simulink model "Scratch_Start"  (R2022a)
settings: Solver=VariableStepAuto  StartTime=0.0  StopTime=inf  RelTol=1e-3
libraries: robotlib x2, simulink x1
settings Model: Creator=dorleco  LastModifiedBy=dorleco

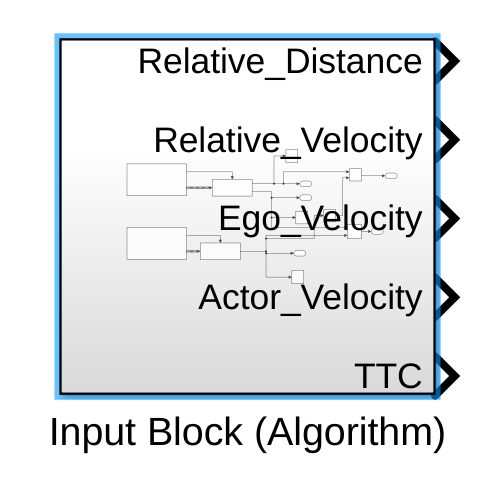
[thumbnail: Simulink's stored preview of the top-level diagram]
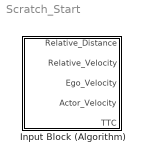
== system Scratch_Start ==
  Input Block (Algorithm) : Subsystem

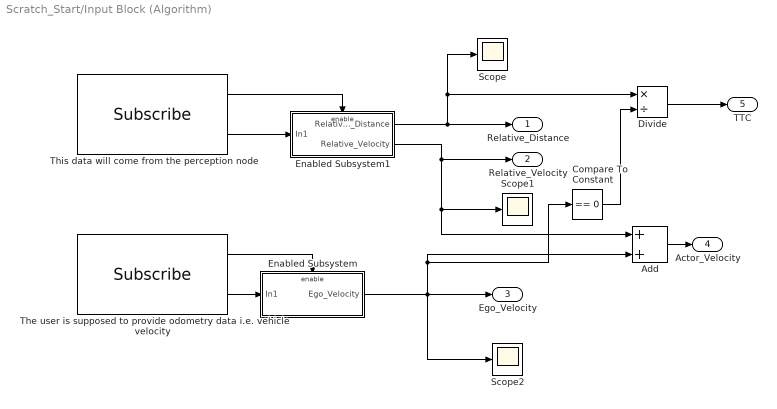
== system Scratch_Start/Input Block (Algorithm) ==
  Add : Sum
  Compare To Constant : simulink/Logic and Bit Operations/Compare To Constant  relop===  const=0  OutDataTypeStr=boolean
  Divide : Product  Inputs=*/
  Enabled Subsystem : Subsystem  TreatAsAtomicUnit=on
  Enabled Subsystem1 : Subsystem  TreatAsAtomicUnit=on
  Scope : Scope
  Scope1 : Scope
  Scope2 : Scope
  The user is supposed to provide odometry data i.e. vehicle velocity : robotlib/Subscribe  topicSource=Select from ROS network  topic=/carla/ego_vehicle/odometry  messageType=nav_msgs/Odometry  SampleTime=0.05  legacyBusStruct=off  messageQueueLength=1
  This data will come from the perception node : robotlib/Subscribe  topicSource=Select from ROS network  topic=/perception/FCW  messageType=geometry_msgs/Point  SampleTime=0.3  legacyBusStruct=off  messageQueueLength=1
  Relative_Distance : Outport
  Relative_Velocity : Outport  Port=2
  Ego_Velocity : Outport  Port=3
  Actor_Velocity : Outport  Port=4
  TTC : Outport  Port=5
  wires:
  Enabled Subsystem1/2(Relative_Velocity) -> Add/1, Scope1/1, Relative_Velocity/1
  This data will come from the perception node/1 -> Enabled Subsystem1/Enable
  This data will come from the perception node/2 -> Enabled Subsystem1/1(In1)
  Enabled Subsystem/1(Ego_Velocity) -> Scope2/1, Ego_Velocity/1, Compare To Constant/1, Add/2
  The user is supposed to provide odometry data i.e. vehicle velocity/1 -> Enabled Subsystem/Enable
  The user is supposed to provide odometry data i.e. vehicle velocity/2 -> Enabled Subsystem/1(In1)
  Enabled Subsystem1/1(Relative_Distance) -> Divide/1, Scope/1, Relative_Distance/1
  Add/1 -> Actor_Velocity/1
  Compare To Constant/1 -> Divide/2
  Divide/1 -> TTC/1

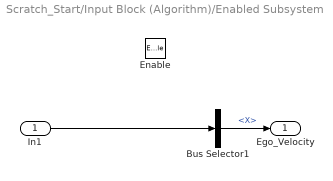
== system Scratch_Start/Input Block (Algorithm)/Enabled Subsystem ==
  In1 : Inport
  Enable : EnablePort
  Bus Selector1 : BusSelector  OutputSignals=Twist.Twist.Linear.X
  Ego_Velocity : Outport
  wires:
  In1/1 -> Bus Selector1/1
  Bus Selector1/1 -> Ego_Velocity/1  "<X>"

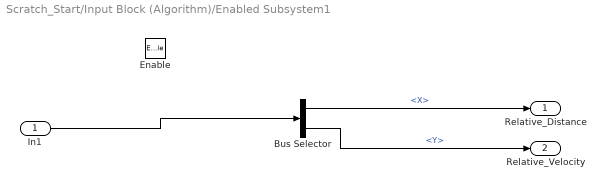
== system Scratch_Start/Input Block (Algorithm)/Enabled Subsystem1 ==
  In1 : Inport
  Enable : EnablePort
  Bus Selector : BusSelector  OutputSignals=X,Y
  Relative_Distance : Outport
  Relative_Velocity : Outport  Port=2
  wires:
  In1/1 -> Bus Selector/1
  Bus Selector/2 -> Relative_Velocity/1  "<Y>"
  Bus Selector/1 -> Relative_Distance/1  "<X>"
